simulink model "Execution_gyro_2_sujet"  (R2018a)
settings: Solver=FixedStepDiscrete  StartTime=0.0  StopTime=inf  RelTol=1e-3  EnableMultiTasking=on
libraries: arduinolib x1
settings Model: SimulationMode=external  ExtModeTrigDuration=2  Creator=Francois  LastModifiedBy=admin-local
settings DataIOCC: LimitDataPoints=on  SaveFormat=Array  SignalLoggingSaveFormat=ModelDataLogs
settings OptimizationCC: EnhancedBackFolding=on  PassReuseOutputArgsAs=Individual arguments  ExpressionDepthLimit=2147483647  MaxStackSize=64  OptimizeBlockOrder=speed  DifferentSizesBufferReuse=on  OptimizationCustomize=off
settings DebuggingCC: UnderspecifiedInitializationDetection=Classic  MergeDetectMultiDrivingBlocksExec=none  SolverPrmCheckMsg=warning  ParameterTunabilityLossMsg=error  FcnCallInpInsideContextMsg=warning  StateNameClashWarn=warning  SFUnexpectedBacktrackingDiag=warning  SFNoUnconditionalDefaultTransitionDiag=warning  SFExecutionAtInitializationDiag=none
settings HardwareCC: ProdBitPerInt=16  ProdBitPerPointer=16  ProdBitPerSizeT=16  ProdBitPerPtrDiffT=16  ProdLargestAtomicFloat=None  ProdWordSize=8  ProdHWDeviceType=Atmel->AVR
settings ModelReferenceCC: PropagateSignalLabelsOutOfModel=off
settings SFSimCC: MATLABDynamicMemAlloc=off
settings RTWCC: SystemTargetFile=ert.tlc  HardwareBoard=Arduino Uno  TLCOptions=-aInlineSetEventsForThisBaseRateFcn=TLC_FALSE -aSuppressMultiTaskScheduler=TLC_FALSE -aRateBasedStepFcn=1  TemplateMakefile=ert_default_tmf  GenerateReport=on  Toolchain=Arduino AVR  BuildConfiguration=Faster Runs  IncludeHyperlinkInReport=on  LaunchReport=on  GenerateTraceInfo=on  GenerateTraceReport=on  GenerateTraceReportSl=on  GenerateTraceReportSf=on  GenerateTraceReportEml=on
settings CodeAppCC: ForceParamTrailComments=on  IgnoreCustomStorageClasses=off  OperatorAnnotations=on  SimulinkDataObjDesc=on  SFDataObjDesc=on  InsertBlockDesc=on
settings ERTTargetCC: SupportContinuousTime=on  SupportVariableSizeSignals=on
settings ConfigComp: CovMetricSettings=dw  CovHtmlReporting=on  CovSaveCumulativeToWorkspaceVar=on  CovSaveSingleToWorkspaceVar=on  CovExternalEMLEnable=off

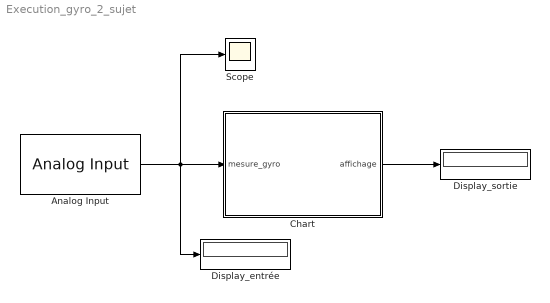
== system Execution_gyro_2_sujet ==
  Analog Input : arduinolib/Analog Input  pinNumber=0  ReadResultsOnly=off  ConversionTriggerSource=Software  ExternalTriggerType=uint32(0)  OutputDataType=uint16  EnableConversionCompleteNotify=off  EnableOuputStatus=off  SampleTime=0.1  blockPlatform=arduino
  Chart : Stateflow chart  TreatAsAtomicUnit=on
  Display_entrée : Display
  Display_sortie : Display
  Scope : Scope
  wires:
  Analog Input/1 -> Chart/1(mesure_gyro), Display_entrée/1, Scope/1
  Chart/1(affichage) -> Display_sortie/1

== stateflow chart Execution_gyro_2_sujet/Chart ==
  state init_compteur
    entry : n = 0 ;
    affichage = n
  state memorise_1
    entry : memo_1 = mesure_gyro
  state memorise_2
    entry : memo_2 = mesure_gyro
  state calcule_ecart
    entry : ecart = memo_2 - memo_1;
    note: A COMPLETER
  note: A COMPLETER
  state init_moyennage
    entry : compte =0;
    moyenne = 0; total = 0
  state memorise_3
    entry : memo_3 = mesure_gyro;
    compte = compte + 1
  note: A COMPLETER
  state calcule_moyenne
    entry :
    affichage = total
    note: A COMPLETER
  state affiche_moyenne
    entry : affichage = moyenne
  (default) -> init_compteur
  init_compteur -> memorise_1 : after(3,sec)
  memorise_1 -> memorise_2 : after(0.1,sec)
  memorise_2 -> calcule_ecart
  init_moyennage -> memorise_3
  memorise_3 -> calcule_moyenne : after(0.1,sec)
  calcule_moyenne -> affiche_moyenne : [compte == 50]
  data: mesure_gyro input; affichage output double; ecart local double; memo_1 local double; memo_2 local double; memo_3 local double; moyenne local double; n local double; compte local double; total local double
